simulink library "Power_Shaft2_Ideal_L1_R1"  (R2024a)
settings: Solver=VariableStepAuto  StartTime=0.0  StopTime=10.0  RelTol=1e-3
undefined symbols (not defined in the file or in its folder): ShaftL1, ShaftR1
libraries: fl_lib x3, Power_Components x2, nesl_utility x2, sm_lib x1
Description:
  | Component of Simscape Vehicle Templates Library
  | 
  | Copyright 2018-2024 The MathWorks, Inc.
settings Model: Creator=smiller  LastModifiedBy=smiller
settings SolverCC: AlgebraicLoopSolver=TrustRegion
settings DataIOCC: ReturnWorkspaceOutputs=off
settings DebuggingCC: UnconnectedInputMsg=warning  UnconnectedOutputMsg=warning  UnconnectedLineMsg=warning  ArithmeticOperatorsInVariantConditions=warning
settings ModelReferenceCC: EnableRefExpFcnMdlSchedulingChecks=on
settings SFSimCC: CustomCodeUndefinedFunction=UseInterfaceOnly
settings RTWCC: GPUComputeCapability=3.5  DLArmComputeVersion=19.05

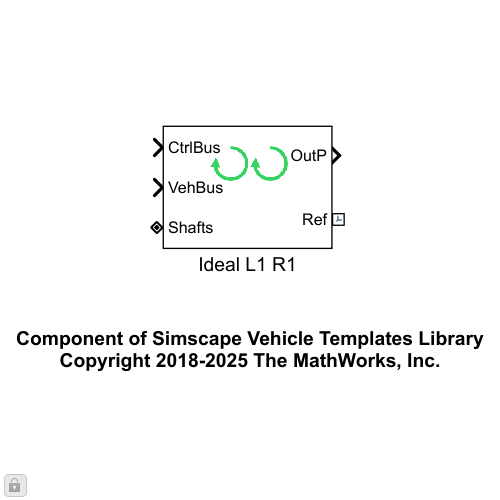
[thumbnail: Simulink's stored preview of the top-level diagram]
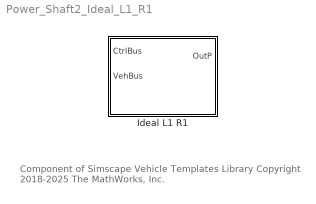
== system Power_Shaft2_Ideal_L1_R1 ==
  note: Component of Simscape Vehicle Templates Library
      | Copyright 2018-2025 The MathWorks, Inc.
  Ideal L1 R1 : Subsystem  VariantControl=IdealTwoMotor  mask(Two Ideal Motors, Left 1 and Right 1){motor_ts_l1=100, motor_ts_r1=100}
      mask prompts: motor_ts_l1 "Left 1 Motor Cutoff Frequency (Hz)"; motor_ts_r1 "Right 1 Motor Cutoff Frequency (Hz)"
      mask help: Models two ideal motors connected to the front left and front right wheels.
      mask Display: image('sm_car_vehicle_power_i2motor_L1R1_IMAGE.png');

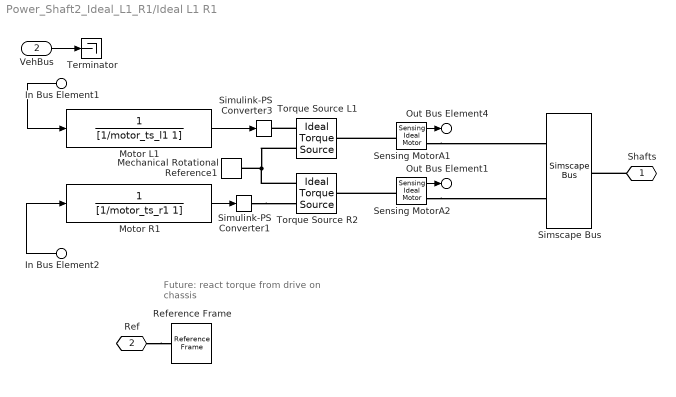
== system Power_Shaft2_Ideal_L1_R1/Ideal L1 R1 ==
  note: Future: react torque from
      | drive on chassis
  In Bus Element1 : Inport  PortName=CtrlBus  Element=MMotorL1Demand
  In Bus Element2 : Inport  PortName=CtrlBus  Element=MMotorR1Demand
  VehBus : Inport  Port=2
  Mechanical Rotational Reference1 : fl_lib/Mechanical/Rotational Elements/Mechanical Rotational Reference
  Motor L1 : TransferFcn  Denominator=[1/motor_ts_l1 1]
  Motor R1 : TransferFcn  Denominator=[1/motor_ts_r1 1]
  Reference Frame : sm_lib/Frames and Transforms/Reference Frame
  Sensing MotorA1 : Power_Components/Sensing Ideal Motor  SystemSampleTime=-1  VariantActivationTime=update diagram  AllowFlexibleInterface=on  Latency=0  AutoFrameSizeCalculation=off
  Sensing MotorA2 : Power_Components/Sensing Ideal Motor  SystemSampleTime=-1  VariantActivationTime=update diagram  AllowFlexibleInterface=on  Latency=0  AutoFrameSizeCalculation=off
  Simscape Bus : SimscapeBus  HierarchyStrings=ShaftL1;ShaftR1
  Simulink-PS Converter1 : nesl_utility/Simulink-PS Converter  PhysicalDomain=network_engine_domain  SubClassName=ps_input  LeftPortType=input  RightPortType=output  PseudoPeriodic=off  Frequencies=[]  NoiseDistribution=none  NoiseParameters=[]  Unit=1  AffineConversion=off  FilteringAndDerivatives=provide  SimscapeFilterOrder=1  InputFilterTimeConstant=0.001  UdotUserProvided=0
  Simulink-PS Converter3 : nesl_utility/Simulink-PS Converter  PhysicalDomain=network_engine_domain  SubClassName=ps_input  LeftPortType=input  RightPortType=output  PseudoPeriodic=off  Frequencies=[]  NoiseDistribution=none  NoiseParameters=[]  Unit=1  AffineConversion=off  FilteringAndDerivatives=provide  SimscapeFilterOrder=1  InputFilterTimeConstant=0.001  UdotUserProvided=0
  Terminator : Terminator
  Torque Source L1 : fl_lib/Mechanical/Mechanical Sources/Ideal Torque Source
  Torque Source R2 : fl_lib/Mechanical/Mechanical Sources/Ideal Torque Source
  Shafts : PMIOPort  Side=Left
  Ref : PMIOPort  Port=2  Side=Right
  Out Bus Element4 : Outport  VectorParamsAs1DForOutWhenUnconnected=off  PortName=OutP  Element=MotorL1
  Out Bus Element1 : Outport  VectorParamsAs1DForOutWhenUnconnected=off  PortName=OutP  Element=MotorR1
  wires:
  Motor R1/1 -> Simulink-PS Converter1/1
  Motor L1/1 -> Simulink-PS Converter3/1
  In Bus Element1/1 -> Motor L1/1
  In Bus Element2/1 -> Motor R1/1
  VehBus/1 -> Terminator/1
  Sensing MotorA1/1 -> Out Bus Element4/1
  Sensing MotorA2/1 -> Out Bus Element1/1
  connections:
  Sensing MotorA2/RConn1 -- Simscape Bus/LConn2
  Sensing MotorA1/RConn1 -- Simscape Bus/LConn1
  Ref/RConn1 -- Reference Frame/RConn1
  Shafts/RConn1 -- Simscape Bus/RConn1
  Torque Source R2/RConn2 -- Mechanical Rotational Reference1/LConn1 -- Torque Source L1/RConn2
  Simulink-PS Converter1/RConn1 -- Torque Source R2/RConn1
  Torque Source L1/RConn1 -- Simulink-PS Converter3/RConn1
  Sensing MotorA1/LConn1 -- Torque Source L1/LConn1
  Sensing MotorA2/LConn1 -- Torque Source R2/LConn1
